simulink model "NFETDemo"  (R2016a)
settings: Solver=VariableStepAuto  StartTime=0.0  StopTime=1  RelTol=1e-3
libraries: fl_lib x7, nesl_utility x3, elec_lib x1
settings Model: Creator=Peter  LastModifiedBy=Peter

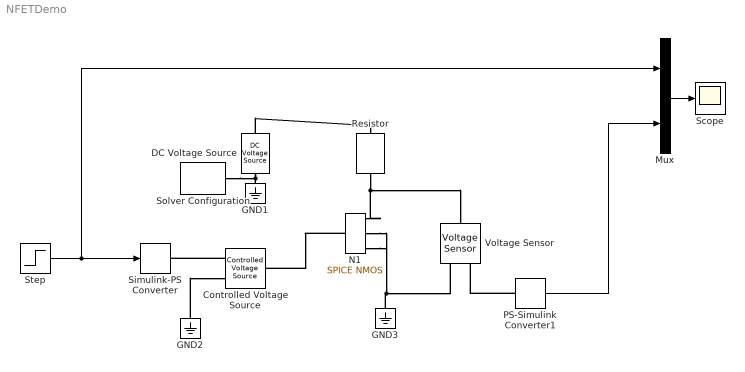
== system NFETDemo ==
  Controlled Voltage Source : fl_lib/Electrical/Electrical Sources/Controlled Voltage Source
  DC Voltage Source : fl_lib/Electrical/Electrical Sources/DC Voltage Source  v0=5 V
  GND1 : fl_lib/Electrical/Electrical Elements/Electrical Reference
  GND2 : fl_lib/Electrical/Electrical Elements/Electrical Reference
  GND3 : fl_lib/Electrical/Electrical Elements/Electrical Reference
  Mux : Mux  Inputs=2
  N1 : elec_lib/Additional Components/SPICE-Compatible Components/Semiconductor Devices/SPICE NMOS  AREA=1  SCALE=1  LENGTH=7.8e-6 m  WIDTH=0.138e-3 m  AD=0.161e-8 m^2  AS=0.603e-8 m^2  PD=0 m  PS=0.478e-3 m  NRD=0.3  NRS=1  LEVEL=1  VTO=0.750 V  KP=NaN A/V^2  GAMMA=1.03 V^0.50000  PHI=0.70 V  LAMBDA=0.018 1/V  RD=NaN Ohm  RS=NaN Ohm  C_param=1  CBD=1e-18 F  CBS=1e-18 F  IS=1.206e-13 A  ND=1  PB=0.9 V  CGSO=0.94e-9 F/m  CGDO=0.59e-9 F/m  CGBO=0.138e-9 F/m  RSH=10 Ohm  CJ=0.39e-3 F/m^2  MJ=0.5  CJSW=264e-12 F/m  MJSW=0.18  JS=20e-6 A/m^2  TOX=0.055e-6 m  LD=1.6e-6 m  U0=650 cm^2/s/V  FC=0.5  NSUB=1e16 1/cm^3  TPG=1  NSS=0.7e11 1/cm^2  UEXP=0  UCRIT=1e+4 V/cm  NEFF=1  DELTA=0  VMAX=1.6e5 m/s  XJ=2.0e-6 m  NFS=1.17e11 1/cm^2  ETA=0  THETA=0 1/V  KAPPA=0.2  T_param=1  TOFFSET=0 K  TFIXED=300.15 K  TMEAS=300.15 K  IC_given=1  ICVDS=0 V  ICVGS=0 V  ICVBS=0 V  MTYPE=1
  PS-Simulink Converter1 : nesl_utility/PS-Simulink Converter  PhysicalDomain=network_engine_domain  SubClassName=ps_output  LeftPortType=input  RightPortType=output  PseudoPeriodic=off  Frequencies=[]  Unit=1  AffineConversion=off
  Resistor : fl_lib/Electrical/Electrical Elements/Resistor  R=10e3 Ohm  i_specify=off  i_priority=None  i=0 A  v_specify=off  v_priority=None  v=0 V
  Scope : Scope
  Simulink-PS Converter : nesl_utility/Simulink-PS Converter  PhysicalDomain=network_engine_domain  SubClassName=ps_input  LeftPortType=input  RightPortType=output  PseudoPeriodic=off  Frequencies=[]  NoiseDistribution=none  NoiseParameters=[]  Unit=V  AffineConversion=off  InputFiltering=on  SimscapeFilterOrder=1  InputFilterTimeConstant=0.001  UdotUserProvided=1
  Solver Configuration : nesl_utility/Solver Configuration  PhysicalDomain=network_engine_domain  SubClassName=solver  LeftPortType=input  RightPortType=generic  Accelerate=off  Tones=[]  Harmonics=[]  SimulateNoise=off  Profile=off  UseLocalSampling=off  EnableSwitchedLinearOptims=on  FrequencyDomain=off  UseCCode=off  RelTol=0.001  AbsTol=1e-06  MinStep=1e-09  ToWorkspace=off  RevertToSquareIcSolve=off  NumHomotopyIterations=100  PhasorMode=off  PhasorModeNumHarmonics=1  OverrideAbsTol=off  DoDC=off  ResidualTolerance=1e-09  UseLocalSolver=off  LocalSolverChoice=NE_BACKWARD_EULER_ADVANCER  LocalSolverSampleTime=0.001  DoFixedCost=off  MaxNonlinIter=3  MaxModeIter=2  LinearAlgebra=Sparse  DelaysMemoryBudget=1024  AutomaticFiltering=on  FilteringTimeConstant=0.001
  Step : Step  Time=.5  After=5  SampleTime=0
  Voltage Sensor : fl_lib/Electrical/Electrical Sensors/Voltage Sensor
  wires:
  PS-Simulink Converter1/1 -> Mux/2
  Mux/1 -> Scope/1
  Step/1 -> Mux/1, Simulink-PS Converter/1
  connections:
  Controlled Voltage Source/RConn1 -- Simulink-PS Converter/RConn1
  GND2/LConn1 -- Controlled Voltage Source/RConn2
  PS-Simulink Converter1/LConn1 -- Voltage Sensor/RConn1
  Resistor/RConn1 -- N1/RConn3 -- Voltage Sensor/LConn1
  GND1/LConn1 -- Solver Configuration/RConn1 -- DC Voltage Source/RConn1
  DC Voltage Source/LConn1 -- Resistor/LConn1
  GND3/LConn1 -- N1/RConn2 -- N1/RConn1 -- Voltage Sensor/RConn2
  N1/LConn1 -- Controlled Voltage Source/LConn1
